simulink model "test_PhaseSep"  (R2015a)
settings: Solver=ode15s  StartTime=0.0  StopTime=1e5  MaxStep=1e2  RelTol=1e-3
libraries: simCryogenics_lib x15, nesl_utility x15
settings Model: Creator=SK248285  LastModifiedBy=SK248285
settings DataIOCC: SaveState=on
settings SimscapeCC: SimscapeLogType=all  SimscapeLogLimitData=off

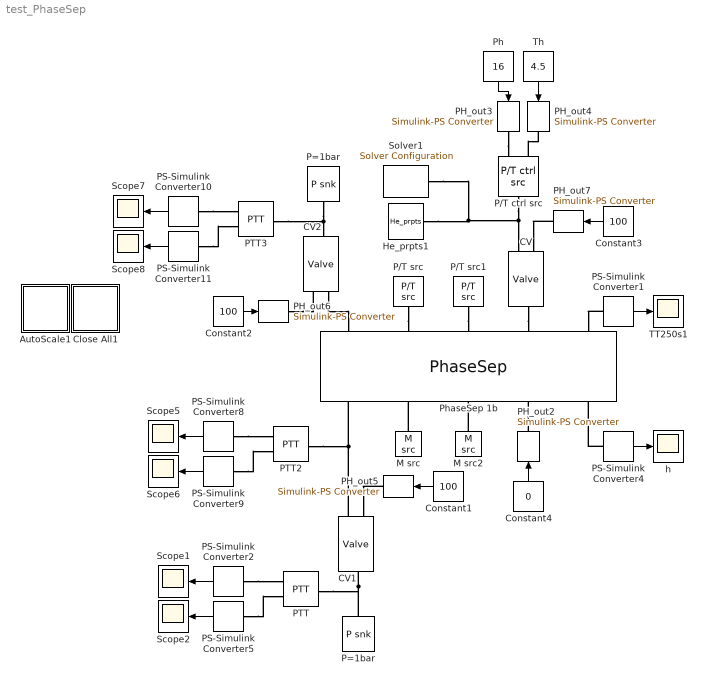
== system test_PhaseSep ==
  AutoScale1 : Subsystem
      settings: OpenFcn=|
      | set(0, 'showhiddenhandles', 'on')
      | 
      | scope = findobj(0, 'Tag', 'SIMULINK_SIMSCOPE_FIGURE');
      | 
      | for i=1:length(scope)
      |   simscope('ScopeBar', 'ActionIcon', 'Find',     scope(i))
      | end
      | 
      | set(0, 'showhiddenhandles', 'off')
      mask Display: disp('Auto\nScale\nScope')
  CV : simCryogenics_lib/Elements/Valve  CVmax=113  ControlInputMin=0  ControlInputMax=100  Xt=0.65  Rv=50  lin_v=0  lim_v=0  K=2.4e-5 m^1.50000*kg^0.50000/s/bar^0.50000  Cmd_specify=off  Cmd_priority=High  Cmd=0  gamma_specify=off  gamma_priority=High  gamma=0  rho_specify=off  rho_priority=High  rho=0 kg/m^3  Xc_specify=off  Xc_priority=High  Xc=0  X_specify=off  X_priority=High  X=0  Y_specify=off  Y_priority=High  Y=0  CV_specify=off  CV_priority=High  CV=0
  CV1 : simCryogenics_lib/Elements/Valve  CVmax=113  ControlInputMin=0  ControlInputMax=100  Xt=0.65  Rv=50  lin_v=0  lim_v=0  K=2.4e-5 m^1.50000*kg^0.50000/s/bar^0.50000  Cmd_specify=off  Cmd_priority=High  Cmd=0  gamma_specify=off  gamma_priority=High  gamma=0  rho_specify=off  rho_priority=High  rho=0 kg/m^3  Xc_specify=off  Xc_priority=High  Xc=0  X_specify=off  X_priority=High  X=0  Y_specify=off  Y_priority=High  Y=0  CV_specify=off  CV_priority=High  CV=0
  CV2 : simCryogenics_lib/Elements/Valve  CVmax=113  ControlInputMin=0  ControlInputMax=100  Xt=0.65  Rv=50  lin_v=0  lim_v=0  K=2.4e-5 m^1.50000*kg^0.50000/s/bar^0.50000  Cmd_specify=off  Cmd_priority=High  Cmd=0  gamma_specify=off  gamma_priority=High  gamma=0  rho_specify=off  rho_priority=High  rho=0 kg/m^3  Xc_specify=off  Xc_priority=High  Xc=0  X_specify=off  X_priority=High  X=0  Y_specify=off  Y_priority=High  Y=0  CV_specify=off  CV_priority=High  CV=0
  Close All1 : Subsystem
      settings: OpenFcn=|
      | set(0, 'showhiddenhandles', 'on')
      | scope = findobj(0, 'Tag','SIMULINK_SIMSCOPE_FIGURE');
      | close(scope)
      | set(0, 'showhiddenhandles', 'off')
      mask Display: disp('Close\nAll\nScope')
  Constant1 : Constant  Value=100
  Constant2 : Constant  Value=100
  Constant3 : Constant  Value=100
  Constant4 : Constant  Value=0
  He_prpts1 : simCryogenics_lib/Utilities/He_prpts  P_min=0.1 bar  T_min=4 K  T_max=320 K  P_max=20 bar  Mol=4.0026 * 10 ^ (- 3) kg/mol
  M src : simCryogenics_lib/Sources_Sinks/M src  M=0 kg/s
  M src2 : simCryogenics_lib/Sources_Sinks/M src  M=0 kg/s
  P/T ctrl src : simCryogenics_lib/Sources_Sinks/P//T ctrl src
  P/T src : simCryogenics_lib/Sources_Sinks/P//T src  P=1.1 bar  T=10 K
  P/T src1 : simCryogenics_lib/Sources_Sinks/P//T src  P=1.1 bar  T=10 K
  P=1bar : simCryogenics_lib/Sources_Sinks/P snk  P=1 bar
  "P=1bar " : simCryogenics_lib/Sources_Sinks/P snk  P=1 bar
  PH_out2 : nesl_utility/Simulink-PS Converter  PhysicalDomain=network_engine_domain  SubClassName=ps_input  LeftPortType=input  RightPortType=output  PseudoPeriodic=off  Frequencies=[]  NoiseDistribution=none  NoiseParameters=[]  Unit=J/s  AffineConversion=off  InputFiltering=on  SimscapeFilterOrder=1  InputFilterTimeConstant=0.001  UdotUserProvided=1
  PH_out{3,5..7} (4 alike) : nesl_utility/Simulink-PS Converter  PhysicalDomain=network_engine_domain  SubClassName=ps_input  LeftPortType=input  RightPortType=output  PseudoPeriodic=off  Frequencies=[]  NoiseDistribution=none  NoiseParameters=[]  Unit=bar  AffineConversion=off  InputFiltering=off  SimscapeFilterOrder=1  InputFilterTimeConstant=0.001  UdotUserProvided=1
  PH_out4 : nesl_utility/Simulink-PS Converter  PhysicalDomain=network_engine_domain  SubClassName=ps_input  LeftPortType=input  RightPortType=output  PseudoPeriodic=off  Frequencies=[]  NoiseDistribution=none  NoiseParameters=[]  Unit=K  AffineConversion=off  InputFiltering=off  SimscapeFilterOrder=1  InputFilterTimeConstant=0.001  UdotUserProvided=1
  PS-Simulink Converter{1..2,4..5,8..11} (8 alike) : nesl_utility/PS-Simulink Converter  PhysicalDomain=network_engine_domain  SubClassName=ps_output  LeftPortType=input  RightPortType=output  PseudoPeriodic=off  Frequencies=[]  Unit=1  AffineConversion=off
  PTT : simCryogenics_lib/Sensors/PTT
  PTT2 : simCryogenics_lib/Sensors/PTT
  PTT3 : simCryogenics_lib/Sensors/PTT
  Ph : Constant  Value=16
  PhaseSep 1b : simCryogenics_lib/Elements/PhaseSep  Ideal1=1  DeltaT1=0.05 K  N1=10  h1=950.3318 W/K  Ideal2=1  DeltaT2=0.05 K  N2=10  h2=950.3318 W/K  hmax=2.1 m  S=1 m^2  P0=1 bar  h0=0  T0=4.5 K
  Scope{1..2,5..8} (6 alike) : Scope
      Scope1 settings: TimeRange=10000  YMin=3  YMax=6
      Scope2 settings: TimeRange=10000  YMin=3  YMax=6
      Scope5 settings: TimeRange=10000  YMin=3  YMax=6  SaveName=ScopeData4
      Scope6 settings: TimeRange=10000  YMin=3  YMax=6  SaveName=ScopeData5
      Scope7 settings: TimeRange=10000  YMin=3  YMax=6  SaveName=ScopeData6
      Scope8 settings: TimeRange=10000  YMin=3  YMax=6  SaveName=ScopeData7
  Solver1 : nesl_utility/Solver Configuration  PhysicalDomain=network_engine_domain  SubClassName=solver  LeftPortType=input  RightPortType=generic  Accelerate=off  Tones=[]  Harmonics=[]  SimulateNoise=off  Profile=off  UseLocalSampling=off  EnableSwitchedLinearOptims=on  FrequencyDomain=off  UseCCode=off  RelTol=0.001  AbsTol=1e-06  MinStep=1e-09  ToWorkspace=off  RevertToSquareIcSolve=off  NumHomotopyIterations=100  DoDC=off  ResidualTolerance=1e-09  UseLocalSolver=off  LocalSolverChoice=NE_BACKWARD_EULER_ADVANCER  LocalSolverSampleTime=5  DoFixedCost=off  MaxNonlinIter=3  MaxModeIter=2  LinearAlgebra=Sparse  DelaysMemoryBudget=1024  AutomaticFiltering=on  FilteringTimeConstant=0.001
  TT250s1 : Scope
      settings: TimeRange=100000  YMin=1  YMax=3  SaveName=TT1
  Th : Constant  Value=4.5
  h : Scope
      settings: TimeRange=100000  YMin=67.1304  YMax=74.1968  SaveName=TT4
  wires:
  Th/1 -> PH_out4/1
  Ph/1 -> PH_out3/1
  PS-Simulink Converter1/1 -> TT250s1/1
  Constant2/1 -> PH_out6/1
  Constant3/1 -> PH_out7/1
  Constant1/1 -> PH_out5/1
  PS-Simulink Converter4/1 -> h/1
  PS-Simulink Converter2/1 -> Scope1/1
  PS-Simulink Converter5/1 -> Scope2/1
  PS-Simulink Converter8/1 -> Scope5/1
  PS-Simulink Converter9/1 -> Scope6/1
  PS-Simulink Converter10/1 -> Scope7/1
  PS-Simulink Converter11/1 -> Scope8/1
  Constant4/1 -> PH_out2/1
  connections:
  PH_out3/RConn1 -- P/T ctrl src/LConn1
  P/T ctrl src/LConn2 -- PH_out4/RConn1
  He_prpts1/RConn1 -- Solver1/RConn1 -- CV/LConn2 -- P/T ctrl src/RConn1
  M src/RConn1 -- PhaseSep 1b/RConn2
  CV1/LConn2 -- PTT2/LConn1 -- PhaseSep 1b/RConn1
  CV2/LConn2 -- PhaseSep 1b/LConn1
  P/T src/RConn1 -- PhaseSep 1b/LConn2
  M src2/RConn1 -- PhaseSep 1b/RConn3
  PS-Simulink Converter1/LConn1 -- PhaseSep 1b/LConn5
  CV/RConn1 -- PhaseSep 1b/LConn4
  P/T src1/RConn1 -- PhaseSep 1b/LConn3
  PH_out6/RConn1 -- CV2/LConn1
  PH_out7/RConn1 -- CV/LConn1
  PH_out5/RConn1 -- CV1/LConn1
  P=1bar/RConn1 -- PTT3/LConn1 -- CV2/RConn1
  CV1/RConn1 -- "P=1bar "/RConn1 -- PTT/LConn1
  PS-Simulink Converter4/LConn1 -- PhaseSep 1b/RConn5
  PS-Simulink Converter2/LConn1 -- PTT/RConn1
  PS-Simulink Converter5/LConn1 -- PTT/RConn2
  PS-Simulink Converter9/LConn1 -- PTT2/RConn2
  PS-Simulink Converter8/LConn1 -- PTT2/RConn1
  PS-Simulink Converter10/LConn1 -- PTT3/RConn1
  PS-Simulink Converter11/LConn1 -- PTT3/RConn2
  PH_out2/RConn1 -- PhaseSep 1b/RConn4

== system test_PhaseSep/AutoScale1 ==

== system test_PhaseSep/Close All1 ==
